simulink model "Car7"  (R2024a)
settings: Solver=VariableStepAuto  StartTime=0.0  StopTime=inf  RelTol=1e-3
model workspace (MAT data in the model file):
  indicator = -1
libraries: arduinolib x1
(part 2 of 2)

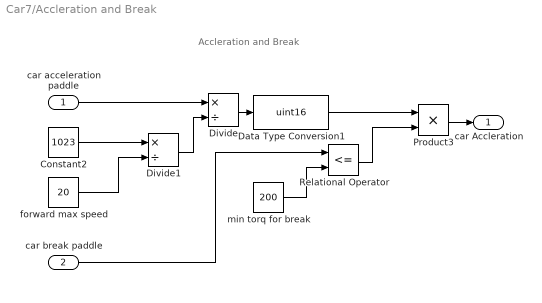
== system Car7/Accleration and Break ==
  note: Accleration and Break
  car acceleration paddle : Inport
  car break paddle : Inport  Port=2
  Constant2 : Constant  Value=1023
  Data Type Conversion1 : DataTypeConversion  OutDataTypeStr=uint16  SaturateOnIntegerOverflow=off  RndMeth=Floor
  Divide : Product  Inputs=*/  RndMeth=Zero  SaturateOnIntegerOverflow=on
  Divide1 : Product  Inputs=*/  RndMeth=Zero  SaturateOnIntegerOverflow=on
  Product3 : Product
  Relational Operator : RelationalOperator  Operator=<=  OutDataTypeStr=boolean  RndMeth=Simplest  InputSameDT=off
  forward max speed : Constant  Value=20
  min torq for break : Constant  Value=200
  car Accleration : Outport
  wires:
  min torq for break/1 -> Relational Operator/2
  Divide/1 -> Data Type Conversion1/1
  forward max speed/1 -> Divide1/2
  car break paddle/1 -> Relational Operator/1
  Data Type Conversion1/1 -> Product3/1
  Constant2/1 -> Divide1/1
  Divide1/1 -> Divide/2
  Relational Operator/1 -> Product3/2
  car acceleration paddle/1 -> Divide/1
  Product3/1 -> car Accleration/1

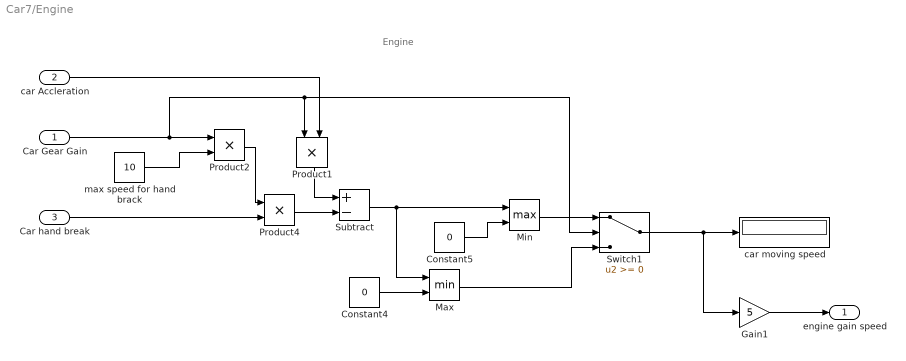
== system Car7/Engine ==
  note: Engine
  Car Gear Gain : Inport
  car Accleration : Inport  Port=2
  "Car hand break " : Inport  Port=3
  Constant4 : Constant  Value=0
  Constant5 : Constant  Value=0
  Gain1 : Gain  Gain=5
  Max : MinMax  Inputs=2
  Min : MinMax  Function=max  Inputs=2
  Product1 : Product
  Product2 : Product
  Product4 : Product
  Subtract : Sum  Inputs=+-
  Switch1 : Switch  SaturateOnIntegerOverflow=off  InputSameDT=off
  car moving speed : Display
  max speed for hand brack : Constant  Value=10
  engine gain speed : Outport
  wires:
  Subtract/1 -> Min/1, Max/1
  Switch1/1 -> Gain1/1, car moving speed/1
  Product2/1 -> Product4/1
  Product1/1 -> Subtract/1
  Product4/1 -> Subtract/2
  Constant5/1 -> Min/2
  max speed for hand brack/1 -> Product2/2
  Car Gear Gain/1 -> Product1/1, Switch1/2, Product2/1
  Max/1 -> Switch1/3
  Min/1 -> Switch1/1
  Constant4/1 -> Max/2
  car Accleration/1 -> Product1/2
  "Car hand break "/1 -> Product4/2
  Gain1/1 -> engine gain speed/1

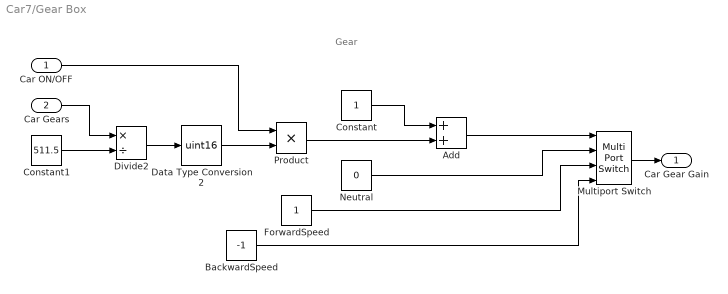
== system Car7/Gear Box ==
  note: Gear
  Car ON/OFF : Inport
  Car Gears : Inport  Port=2
  Add : Sum
  BackwardSpeed : Constant  Value=-1
  Constant : Constant
  Constant1 : Constant  Value=511.5
  Data Type Conversion2 : DataTypeConversion  OutDataTypeStr=uint16  RndMeth=Nearest  SaturateOnIntegerOverflow=off
  Divide2 : Product  Inputs=*/  RndMeth=Zero  SaturateOnIntegerOverflow=on
  ForwardSpeed : Constant
  Multiport Switch : MultiPortSwitch  SaturateOnIntegerOverflow=off  InputSameDT=off
  Neutral : Constant  Value=0
  Product : Product
  Car Gear Gain : Outport
  wires:
  Add/1 -> Multiport Switch/1
  Neutral/1 -> Multiport Switch/2
  Constant1/1 -> Divide2/2
  Product/1 -> Add/2
  BackwardSpeed/1 -> Multiport Switch/4
  Data Type Conversion2/1 -> Product/2
  ForwardSpeed/1 -> Multiport Switch/3
  Divide2/1 -> Data Type Conversion2/1
  Constant/1 -> Add/1
  Car Gears/1 -> Divide2/1
  Multiport Switch/1 -> Car Gear Gain/1
  Car ON/OFF/1 -> Product/1

== matlab function Car7/MATLAB Function ==
  data: u input; y output
function y = fcn(u)

y = u;
